simulink library "Lib_Thermo_Enth2Temp_TMATS"  (R2013b)
settings: Solver=ode45  StartTime=0.0  StopTime=10.0  RelTol=1e-3
Description:
  | Thomas Modules
settings Model: Creator=jwchapm2  LastModifiedBy=jwchapm2

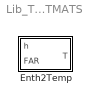
== system Lib_Thermo_Enth2Temp_TMATS ==
  Enth2Temp : Subsystem  mask(T-MATS: Enth2Temp Library Block){}
      mask help: This block emperically calculates temperature (T) from enthalpy (h) and fuel to air ratio (FAR).
      mask Help: web(which('Thermo_TMATS_Enth2Temp.html'),'-helpbrowser')

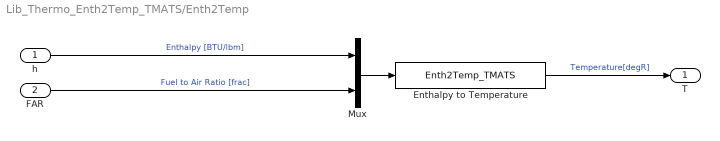
== system Lib_Thermo_Enth2Temp_TMATS/Enth2Temp ==
  h : Inport
  FAR : Inport  Port=2
  "Enthalpy to Temperature " : S-Function  FunctionName=Enth2Temp_TMATS  EnableBusSupport=off
  Mux : Mux  Inputs=2
  T : Outport
  wires:
  "Enthalpy to Temperature "/1 -> T/1  "Temperature[degR]"
  Mux/1 -> "Enthalpy to Temperature "/1
  h/1 -> Mux/1  "Enthalpy [BTU/lbm]"
  FAR/1 -> Mux/2  "Fuel to Air Ratio [frac]"
